simulink model "signalClassification"  (R2020a)
settings: Solver=ode45  StartTime=0.0  StopTime=Tf  RelTol=1e-3  EnableMultiTasking=on
libraries: simulink x4, rllib x1
settings Model: Creator=The MathWorks, Inc.  LastModifiedBy=DELL
settings DataIOCC: LimitDataPoints=on  SaveFormat=Array  SignalLoggingName=logsOut
settings OptimizationCC: ExpressionDepthLimit=2147483647  InitFltsAndDblsToZero=on  LifeSpan=inf
settings DebuggingCC: SaveWithParameterizedLinksMsg=none  UnderspecifiedInitializationDetection=Classic  MergeDetectMultiDrivingBlocksExec=none  SignalResolutionControl=TryResolveAllWithWarning  MultiTaskDSMMsg=warning  FcnCallInpInsideContextMsg=warning  AllowSymbolicDim=off  StateNameClashWarn=warning  SFUnexpectedBacktrackingDiag=warning  SFNoUnconditionalDefaultTransitionDiag=warning  SFExecutionAtInitializationDiag=none  ArithmeticOperatorsInVariantConditions=warning
settings HardwareCC: ProdBitPerPointer=32  ProdBitPerSizeT=32  ProdBitPerPtrDiffT=32  ProdLargestAtomicFloat=None  ProdIntDivRoundTo=Undefined  ProdEndianess=Unspecified  ProdWordSize=32  ProdHWDeviceType=Specified
settings ModelReferenceCC: PropagateSignalLabelsOutOfModel=off
settings SFSimCC: SimUseLocalCustomCode=off
settings RTWCC: RTWUseLocalCustomCode=off
settings CodeAppCC: StateflowObjectComments=on
settings GRTTargetCC: TargetFcnLib=ansi_tfl_tmw.mat  TargetLangStandard=C89/C90 (ANSI)  CombineOutputUpdateFcns=off  GRTInterface=on
settings ConfigComp: CovMetricSettings=dw  CovHtmlReporting=on  CovSaveCumulativeToWorkspaceVar=on  CovSaveSingleToWorkspaceVar=on  CovExternalEMLEnable=off

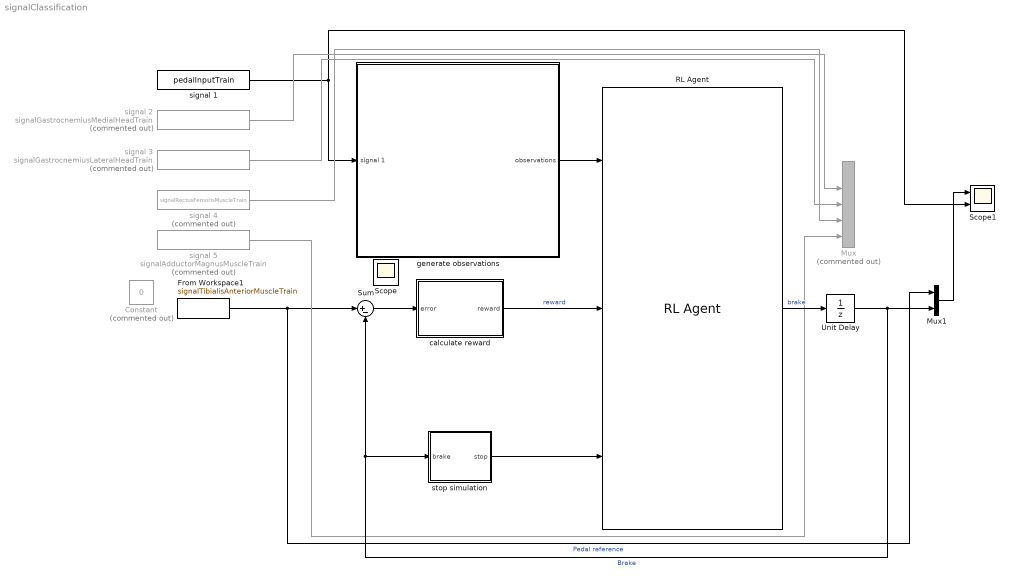
== system signalClassification ==
  Constant : Constant  Commented=on  Value=0
  From Workspace1 : FromWorkspace  VariableName=signalTibialisAnteriorMuscleTrain
  Mux : Mux  Commented=on  Inputs=5
  Mux1 : Mux  Inputs=2
  RL Agent : rllib/RL Agent  Agent=agent  ProvideReward=on  ProvideIsDone=on  ProvideCumRwd=off  TreatAsDirectFeedthrough=on  CollectLoggedSignals=on  CollectModelStates=on
  Scope1 : Scope  NumInputPorts=2
  Sum : Sum  Inputs=|+-
  Unit Delay : UnitDelay  SampleTime=0.01  HasFrameUpgradeWarning=on
  calculate reward : Subsystem
  generate observations : Subsystem
  signal 1 : FromWorkspace  VariableName=pedalInputTrain
  signal 2 : FromWorkspace  Commented=on  VariableName=signalGastrocnemiusMedialHeadTrain
  signal 3 : FromWorkspace  Commented=on  VariableName=signalGastrocnemiusLateralHeadTrain
  signal 4 : FromWorkspace  Commented=on  VariableName=signalRectusFemorisMuscleTrain
  signal 5 : FromWorkspace  Commented=on  VariableName=signalAdductorMagnusMuscleTrain
  stop simulation : Subsystem
  Scope : Scope
  wires:
  signal 1/1 -> Scope1/2, generate observations/1(signal 1)
  stop simulation/1(stop) -> RL Agent/3
  calculate reward/1(reward) -> RL Agent/2  "reward"
  generate observations/1(observations) -> RL Agent/1
  From Workspace1/1 -> Mux1/1, Sum/1  "Pedal reference"
  Sum/1 -> calculate reward/1(error)
  signal 2/1 -> Mux/2
  signal 3/1 -> Mux/3
  signal 4/1 -> Mux/4
  signal 5/1 -> Mux/5
  RL Agent/1 -> Unit Delay/1  "brake"
  Unit Delay/1 -> Sum/2, stop simulation/1(brake), Mux1/2  "Brake"
  Mux1/1 -> Scope1/1

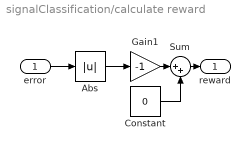
== system signalClassification/calculate reward ==
  error : Inport
  Abs : Abs
  Constant : Constant  Value=0
  Gain1 : Gain  Gain=-1
  Sum : Sum  Inputs=|++
  reward : Outport  VectorParamsAs1DForOutWhenUnconnected=off
  wires:
  Abs/1 -> Gain1/1
  error/1 -> Abs/1
  Sum/1 -> reward/1
  Gain1/1 -> Sum/1
  Constant/1 -> Sum/2

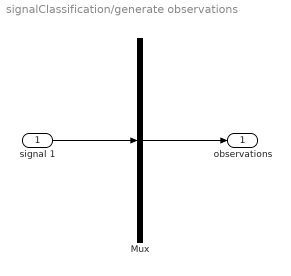
== system signalClassification/generate observations ==
  signal 1 : Inport
  Mux : Mux  Inputs=1
  observations : Outport  VectorParamsAs1DForOutWhenUnconnected=off
  wires:
  signal 1/1 -> Mux/1
  Mux/1 -> observations/1

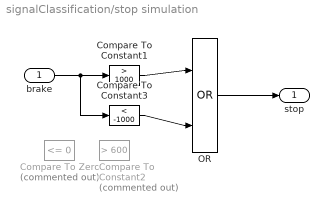
== system signalClassification/stop simulation ==
  brake : Inport
  Compare To Constant1 : simulink/Logic and Bit Operations/Compare To Constant  relop=>  const=1000  OutDataTypeStr=boolean
  Compare To Constant2 : simulink/Logic and Bit Operations/Compare To Constant  Commented=on  relop=>  const=600  OutDataTypeStr=boolean
  Compare To Constant3 : simulink/Logic and Bit Operations/Compare To Constant  relop=<  const=-1000  OutDataTypeStr=boolean
  Compare To Zero : simulink/Logic and Bit Operations/Compare To Zero  Commented=on  relop=<=  OutDataTypeStr=boolean
  OR : Logic  Operator=OR  IconShape=distinctive  AllPortsSameDT=off  OutDataTypeStr=boolean
  stop : Outport  VectorParamsAs1DForOutWhenUnconnected=off
  wires:
  brake/1 -> Compare To Constant3/1, Compare To Constant1/1
  Compare To Constant3/1 -> OR/2
  Compare To Constant1/1 -> OR/1
  OR/1 -> stop/1
